simulink model "mux_demux_ex1"  (R2021a)
settings: Solver=VariableStepAuto  StartTime=0.0  StopTime=10.0  RelTol=1e-3
settings Model: Creator=lenovo  LastModifiedBy=lenovo

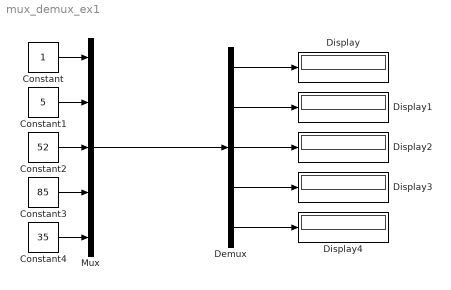
== system mux_demux_ex1 ==
  Constant : Constant
  Constant1 : Constant  Value=5
  Constant2 : Constant  Value=52
  Constant3 : Constant  Value=85
  Constant4 : Constant  Value=35
  Demux : Demux  Outputs=5
  Display{,1..4} (5 alike) : Display
  Mux : Mux  Inputs=5
  wires:
  Constant1/1 -> Mux/2
  Constant2/1 -> Mux/3
  Constant3/1 -> Mux/4
  Constant4/1 -> Mux/5
  Constant/1 -> Mux/1
  Mux/1 -> Demux/1
  Demux/1 -> Display/1
  Demux/2 -> Display1/1
  Demux/3 -> Display2/1
  Demux/4 -> Display3/1
  Demux/5 -> Display4/1
